simulink model "AM_DSB_LC_DEMODULATION"  (R2024a)
settings: Solver=VariableStepAuto  StartTime=0.0  StopTime=10.0  RelTol=1e-3
libraries: dspfdesign x1
settings Model: Creator=zeyad  LastModifiedBy=zeyad

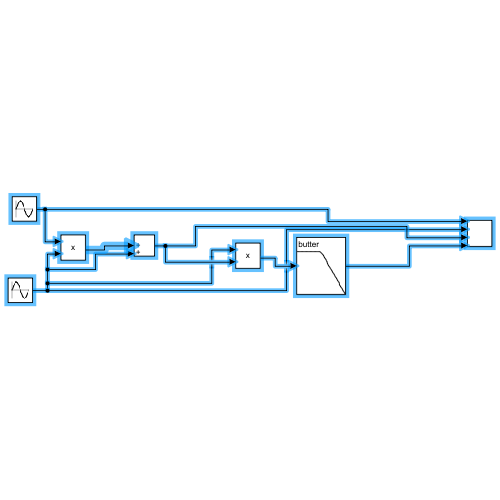
[thumbnail: Simulink's stored preview of the top-level diagram]
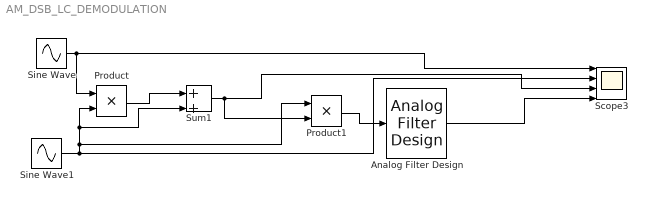
== system AM_DSB_LC_DEMODULATION ==
  Analog Filter Design : dspfdesign/Analog Filter Design  method=Butterworth  filttype=Lowpass  N=8  Wlo=60  Whi=80  Rp=2  Rs=40
  Product : Product
  Product1 : Product
  Scope3 : Scope  NumInputPorts=4
  Sine Wave : Sin  Frequency=5  SampleTime=0
  Sine Wave1 : Sin  Frequency=50  SampleTime=0
  Sum1 : Sum  Inputs=|++
  wires:
  Analog Filter Design/1 -> Scope3/4
  Sine Wave/1 -> Scope3/1, Product/1
  Sine Wave1/1 -> Scope3/2, Product1/1, Sum1/2, Product/2
  Product1/1 -> Analog Filter Design/1
  Sum1/1 -> Product1/2, Scope3/3
  Product/1 -> Sum1/1
